simulink model "souk_single_pipeline_4x2"  (R2021a)
settings: Solver=VariableStepAuto  StartTime=0.0  StopTime=10.0  RelTol=1e-3
undefined symbols (not defined in the file): datetime, posixtime
libraries: xbsIndex_r4 x9016, casper_library_misc x75, casper_library_delays x33, casper_library_reorder x22, xps_library x10
(part 35 of 104)

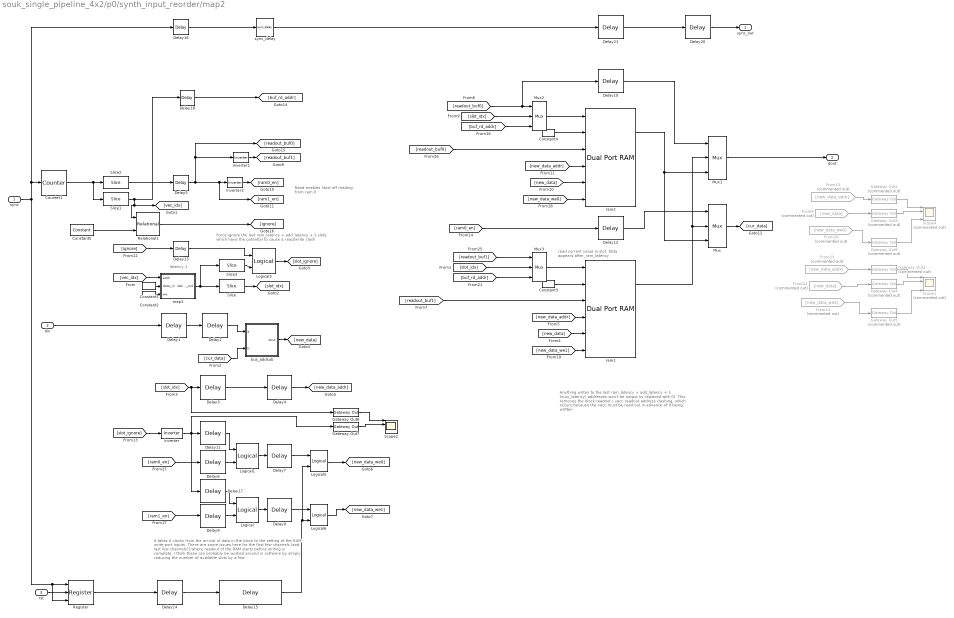
== system souk_single_pipeline_4x2/p0/synth_input_reorder/map2 ==
  note: latency 1
  note: read current value in slot.
      | Data appears after_ram_latency
  note: Read enables
      | Start off reading from ram 0
  note: It takes 6 clocks from the arrival of data in the block
      | to the setting of the RAM write-port inputs. There are some issues
      | here for the first few channels (and last few channels?) where readout
      | of the RAM starts before writing is complete. I think these can probably
      | be worked around in software by simply reducing the number of available
      | slots by a few
  note: Anything writen to the last
      | ram_latency + add_latency + 1 (mux_latency)
      | addresses won't be output (is replaced with 0).
      | This removes the block readout / vacc readout address clashing,
      | which occurs because the vacc must be read out in advance of
      | it being written
  note: Force ignore the last ram_latency + add_latency + 1 slots,
      | which have the potential to cause a read/write clash
  sync : Inport
  din : Inport  Port=2
  rst : Inport  Port=3
  Constant1 : xbsIndex_r4/Constant  const=0  gui_display_data_type=Fixed-point  arith_type=Unsigned  n_bits=32  bin_pt=0  preci_type=Single  exp_width=8  frac_width=24  explicit_period=on  period=1  equ=P=C  opselect=C  inp2=PCIN>>17  opr=+  inp1=P  carry=CIN  dbl_ovrd=off  block_type=constant
  Constant2 : xbsIndex_r4/Constant  const=0  gui_display_data_type=Boolean  arith_type=Boolean  n_bits=32  bin_pt=0  preci_type=Single  exp_width=8  frac_width=24  explicit_period=on  period=1  equ=P=C  opselect=C  inp2=PCIN>>17  opr=+  inp1=P  carry=CIN  dbl_ovrd=off  block_type=constant
  Constant3 : xbsIndex_r4/Constant  const=0  gui_display_data_type=Fixed-point  arith_type=Unsigned  n_bits=2*sample_width * n_samples  bin_pt=0  preci_type=Single  exp_width=8  frac_width=24  explicit_period=on  period=1  equ=P=C  opselect=C  inp2=PCIN>>17  opr=+  inp1=P  carry=CIN  dbl_ovrd=off  block_type=constant
  Constant4 : xbsIndex_r4/Constant  const=0  gui_display_data_type=Fixed-point  arith_type=Unsigned  n_bits=2*sample_width * n_samples  bin_pt=0  preci_type=Single  exp_width=8  frac_width=24  explicit_period=on  period=1  equ=P=C  opselect=C  inp2=PCIN>>17  opr=+  inp1=P  carry=CIN  dbl_ovrd=off  block_type=constant
  Constant5 : xbsIndex_r4/Constant  const="(2^vec_len_bits - 1) - (ram_latency + add_latency +  1 + 1 + 1)"  gui_display_data_type=Fixed-point  arith_type=Unsigned  n_bits=vec_len_bits  bin_pt=0  preci_type=Single  exp_width=8  frac_width=24  explicit_period=on  period=1  equ=P=C  opselect=C  inp2=PCIN>>17  opr=+  inp1=P  carry=CIN  dbl_ovrd=off  block_type=constant
  Counter1 : xbsIndex_r4/Counter  cnt_type=Free Running  cnt_to=Inf  operation=Up  start_count=0  cnt_by_val=1  arith_type=Unsigned  n_bits=vec_len_bits + 1  bin_pt=0  load_pin=off  rst=on  en=off  explicit_period=on  period=1  use_behavioral_HDL=off  implementation=Fabric  dbl_ovrd=off  block_type=counter
  Delay{1,5..6,8,13..14,16,18,20} (9 alike) : xbsIndex_r4/Delay  rst=off  infoeditControl=Selection of Reset will increase slice count due to use of real FFs and instead of SRLs  en=off  latency=1  reg_retiming=on  dbl_ovrd=off  block_type=delay
  Delay10 : xbsIndex_r4/Delay  rst=off  infoeditControl=Selection of Reset will increase slice count due to use of real FFs and instead of SRLs  en=off  latency=ram_latency  reg_retiming=on  dbl_ovrd=off  block_type=delay
  Delay11 : xbsIndex_r4/Delay  rst=off  infoeditControl=Selection of Reset will increase slice count due to use of real FFs and instead of SRLs  en=off  latency=1  reg_retiming=off  dbl_ovrd=off  block_type=delay
  Delay12 : xbsIndex_r4/Delay  rst=off  infoeditControl=Selection of Reset will increase slice count due to use of real FFs and instead of SRLs  en=off  latency=ram_latency  reg_retiming=on  dbl_ovrd=off  block_type=delay
  Delay15 : xbsIndex_r4/Delay  rst=off  infoeditControl=Selection of Reset will increase slice count due to use of real FFs and instead of SRLs  en=off  latency=ram_latency + add_latency +1  reg_retiming=on  dbl_ovrd=off  block_type=delay
  Delay17 : xbsIndex_r4/Delay  rst=off  infoeditControl=Selection of Reset will increase slice count due to use of real FFs and instead of SRLs  en=off  latency=1  reg_retiming=off  dbl_ovrd=off  block_type=delay
  Delay2 : xbsIndex_r4/Delay  rst=off  infoeditControl=Selection of Reset will increase slice count due to use of real FFs and instead of SRLs  en=off  latency=ram_latency+1  reg_retiming=on  dbl_ovrd=off  block_type=delay
  Delay21 : xbsIndex_r4/Delay  rst=off  infoeditControl=Selection of Reset will increase slice count due to use of real FFs and instead of SRLs  en=off  latency=ram_latency  reg_retiming=on  dbl_ovrd=off  block_type=delay
  Delay3 : xbsIndex_r4/Delay  rst=off  infoeditControl=Selection of Reset will increase slice count due to use of real FFs and instead of SRLs  en=off  latency=ram_latency+1  reg_retiming=on  dbl_ovrd=off  block_type=delay
  Delay4 : xbsIndex_r4/Delay  rst=off  infoeditControl=Selection of Reset will increase slice count due to use of real FFs and instead of SRLs  en=off  latency=add_latency  reg_retiming=on  dbl_ovrd=off  block_type=delay
  Delay7 : xbsIndex_r4/Delay  rst=off  infoeditControl=Selection of Reset will increase slice count due to use of real FFs and instead of SRLs  en=off  latency=add_latency  reg_retiming=on  dbl_ovrd=off  block_type=delay
  Delay9 : xbsIndex_r4/Delay  rst=off  infoeditControl=Selection of Reset will increase slice count due to use of real FFs and instead of SRLs  en=off  latency=add_latency  reg_retiming=on  dbl_ovrd=off  block_type=delay
  From15 : From  Commented=on  GotoTag=new_data_addr
  From20 : From  Commented=on  GotoTag=new_data_we0
  From22 : From  Commented=on  GotoTag=new_data
  From23 : From  Commented=on  GotoTag=new_data_addr
  From24 : From  Commented=on  GotoTag=new_data_we1
  From8 : From  Commented=on  GotoTag=new_data
  Gateway Out{1..5,9} (6 alike) : xbsIndex_r4/Gateway Out  Commented=on  inherit_from_input=off  hdl_port=off  rows=1  columns=1  UseAsDAC=off  DACChannel='1'  interface=None  automatic_assignment=on  address_offset=hex2dec('00')  intf_name=''  intf_description=''  timing_constraint=None  locs_specified=off  LOCs={}  io_standard={}  block_type=gatewayout
  Gateway Out6 : xbsIndex_r4/Gateway Out  inherit_from_input=off  hdl_port=off  rows=1  columns=1  UseAsDAC=off  DACChannel='1'  interface=None  automatic_assignment=on  address_offset=hex2dec('00')  intf_name=''  intf_description=''  timing_constraint=None  locs_specified=off  LOCs={}  io_standard={}  block_type=gatewayout
  Gateway Out7 : xbsIndex_r4/Gateway Out  inherit_from_input=off  hdl_port=off  rows=1  columns=1  UseAsDAC=off  DACChannel='1'  interface=None  automatic_assignment=on  address_offset=hex2dec('00')  intf_name=''  intf_description=''  timing_constraint=None  locs_specified=off  LOCs={}  io_standard={}  block_type=gatewayout
  Inverter : xbsIndex_r4/Inverter  en=off  latency=0  dbl_ovrd=off  block_type=inv
  Inverter1 : xbsIndex_r4/Inverter  en=off  latency=0  dbl_ovrd=off  block_type=inv
  Inverter3 : xbsIndex_r4/Inverter  en=off  latency=0  dbl_ovrd=off  block_type=inv
  Logical : xbsIndex_r4/Logical  logical_function=AND  inputs=2  en=off  latency=ram_latency  precision=Full  arith_type=Unsigned  n_bits=16  bin_pt=0  align_bp=on  dbl_ovrd=off  block_type=logical
  Logical1 : xbsIndex_r4/Logical  logical_function=AND  inputs=2  en=off  latency=ram_latency  precision=Full  arith_type=Unsigned  n_bits=16  bin_pt=0  align_bp=on  dbl_ovrd=off  block_type=logical
  Logical3 : xbsIndex_r4/Logical  logical_function=OR  inputs=2  en=off  latency=0  precision=Full  arith_type=Unsigned  n_bits=16  bin_pt=0  align_bp=on  dbl_ovrd=off  block_type=logical
  Logical5 : xbsIndex_r4/Logical  logical_function=AND  inputs=2  en=off  latency=0  precision=Full  arith_type=Unsigned  n_bits=16  bin_pt=0  align_bp=on  dbl_ovrd=off  block_type=logical
  Logical6 : xbsIndex_r4/Logical  logical_function=AND  inputs=2  en=off  latency=0  precision=Full  arith_type=Unsigned  n_bits=16  bin_pt=0  align_bp=on  dbl_ovrd=off  block_type=logical
  Mux : xbsIndex_r4/Mux  inputs=2  en=off  latency=1  precision=Full  arith_type=Unsigned  n_bits=16  bin_pt=14  quantization=Truncate  overflow=Wrap  dbl_ovrd=off  block_type=mux
  Mux1 : xbsIndex_r4/Mux  inputs=2  en=off  latency=1  precision=Full  arith_type=Unsigned  n_bits=16  bin_pt=14  quantization=Truncate  overflow=Wrap  dbl_ovrd=off  block_type=mux
  Mux2 : xbsIndex_r4/Mux  inputs=2  en=off  latency=0  precision=Full  arith_type=Unsigned  n_bits=16  bin_pt=14  quantization=Truncate  overflow=Wrap  dbl_ovrd=off  block_type=mux
  Mux3 : xbsIndex_r4/Mux  inputs=2  en=off  latency=0  precision=Full  arith_type=Unsigned  n_bits=16  bin_pt=14  quantization=Truncate  overflow=Wrap  dbl_ovrd=off  block_type=mux
  Register : xbsIndex_r4/Register  init=0  rst=on  en=on  dbl_ovrd=off  block_type=register
  Relational1 : xbsIndex_r4/Relational  mode=a>b  op_type=Bool  en=off  latency=0  dbl_ovrd=off  block_type=relational
  Scope1 : Scope  Commented=on  NumInputPorts=4
  Scope2 : Scope  NumInputPorts=4
  Scope4 : Scope  Commented=on  NumInputPorts=4
  Slice : xbsIndex_r4/Slice  nbits=vec_len_bits  boolean_output=off  mode=Lower Bit Location + Width  bit1=0  base1=MSB of Input  bit0=0  base0=LSB of Input  dbl_ovrd=off  block_type=slice
  Slice1 : xbsIndex_r4/Slice  nbits=vec_len_bits  boolean_output=off  mode=Lower Bit Location + Width  bit1=0  base1=MSB of Input  bit0=0  base0=LSB of Input  dbl_ovrd=off  block_type=slice
  Slice2 : xbsIndex_r4/Slice  nbits=1  boolean_output=on  mode=Lower Bit Location + Width  bit1=0  base1=MSB of Input  bit0=vec_len_bits  base0=LSB of Input  dbl_ovrd=off  block_type=slice
  Slice3 : xbsIndex_r4/Slice  nbits=1  boolean_output=on  mode=Upper Bit Location + Width  bit1=0  base1=MSB of Input  bit0=0  base0=LSB of Input  dbl_ovrd=off  block_type=slice
  bus_addsub : Subsystem  AncestorBlock=casper_library_bus/bus_addsub  mask(bus_addsub){opmode=0, n_bits_a=sample_width*ones(n_samples,1), bin_pt_a=zeros(n_samples,1), type_a=1, n_bits_b=sample_width*ones(n_samples,1), bin_pt_b=zeros(n_samples,1), type_b=1, cmplx=on, misc=off, async=off, floating_point=off, float_type=single, exp_width=6, frac_width=19, n_bits_out=sample_width*ones(n_samples,1), bin_pt_out=zeros(n_samples,1), type_out=1, quantization=0, overflow=1, add_implementation=behavioral HDL, csp_latency=add_latency, pipeline_en=off, pipeline_latency=0}
      mask prompts: opmode "mode (Addition=0, Subtraction=1)"; n_bits_a "a input bit widths"; bin_pt_a "a input binary points"; type_a "a input type (Unsigned=0, Signed=1)"; n_bits_b "b input bit widths"; bin_pt_b "b input binary points"; type_b "b input type (Unsigned=0, Signed=1)"; cmplx "complex"; misc "misc support"; async "asynchronous operation"; floating_point "floating point"; exp_width "exponent width"; frac_width "fraction width"; n_bits_out "output bit widths"; bin_pt_out "output binary points"; type_out "output type (Unsigned=0, Signed=1)"; quantization "quantization strategy (Truncate=0, Round  (unbiased: +/- Inf)=1)"; overflow "overflow strategy (Wrap=0, Saturate=1, Flag as error=2)"; add_implementation "adder implementation"; csp_latency "latency"; pipeline_en "pipeline enable"; pipeline_latency "pipeline latency"
      mask help: Add/subtract components of two busses
      mask init: same as souk_single_pipeline_4x2/p0/bus_addsub
      mask Callback floating_point:
      | onoff = get_param(gcb, 'floating_point');
      | if strcmp(onoff,'on')
      |     enable_fixpt = 'off';
      |     set_param_state(gcb, 'float_type', 'on')
      | 
      |     f_type = get_param(gcb, 'float_type');
      |     if strcmp(f_type,'custom')
      |         set_param_state(gcb, 'exp_width', 'on')
      |         set_param_state(gcb, 'frac_width', 'on')
      |     else
      |         set_param_state(gcb, 'exp_width', 'off')
      |         set_param_state(gcb, 'frac_width', 'off')
      |     end
      | 
      | 
      | else
      |     enable_fixpt = 'on';
      |     set_param_state(gcb, 'float_type', 'off')
      |     set_param_state(gcb, 'exp_width', 'off')
      |     set_param_state(gcb, 'frac_width', 'off')
      | end
      | 
      | set_param_state(gcb, 'n_bits_a', enable_fixpt)
      | set_param_state(gcb, 'bin_pt_a', enable_fixpt)
      | set_param_state(gcb, 'type_a', enable_fixpt)
      | set_param_state(gcb, 'n_bits_b', enable_fixpt)
      | set_param_state(gcb, 'bin_pt_b', enable_fixpt)
      | set_param_state(gcb, 'type_b', enable_fixpt)
      | 
      | set_param_state(gcb, 'n_bits_out', enable_fixpt)
      | set_param_state(gcb, 'bin_pt_out', enable_fixpt)
      | set_param_state(gcb, 'type_out', enable_fixpt)
      | set_param_state(gcb, 'quantization', enable_fixpt)
      | set_param_state(gcb, 'overflow', enable_fixpt)
      mask TypeOptions float_type: single | custom
      mask Callback float_type:
      | f_type = get_param(gcb, 'float_type');
      | if strcmp(f_type,'custom')
      |     set_param_state(gcb, 'exp_width', 'on')
      |     set_param_state(gcb, 'frac_width', 'on')
      | else
      |     set_param_state(gcb, 'exp_width', 'off')
      |     set_param_state(gcb, 'frac_width', 'off')
      | end
      mask TypeOptions add_implementation: behavioral HDL | fabric core | DSP48 core
  map1 : Subsystem  Tag=xps:bram  AncestorBlock=xps_library/Memory/shared_bram  mask{arith_type=Unsigned, addr_width=vec_len_bits, data_width=16, reg_prim_output=off, reg_core_output=off, optimization=Minimum_Area, data_bin_pt=0, init_vals=[2^vec_len_bits-1:-1:0], sample_rate=1, desc_str="", type_desc='uint32'}
      mask prompts: arith_type "Output Data Type"; addr_width "Address width"; data_width "Data Width"; reg_prim_output "Register Primitive Output"; reg_core_output "Register Core Output"; data_bin_pt "Data Binary Point"; init_vals "Initial values (simulation only)"; sample_rate "Sample rate"; desc_str "Description"; type_desc "Data Type Description"
      mask init:
      | shared_bram_mask;
      mask TypeOptions arith_type: Unsigned | Signed  (2's comp)
      mask TypeOptions data_width: 8 | 16 | 32 | 64 | 128 | 256 | 512 | 1024
      mask TypeOptions optimization: Minimum_Area | Low_Power
  ram1 : xbsIndex_r4/Dual Port RAM  depth=2^vec_len_bits  initVector=zeros(1,2^vec_len_bits)  distributed_mem=Block RAM  init_a=0  init_b=0  rst_a=off  rst_b=off  en_a=off  en_b=off  latency=ram_latency  write_mode_A=Read Before Write  write_mode_B=Read Before Write  optimize=Area  dbl_ovrd=off  simulation_type=fast_sim  block_type=dpram
  ram2 : xbsIndex_r4/Dual Port RAM  depth=2^vec_len_bits  initVector=zeros(1,2^vec_len_bits)  distributed_mem=Block RAM  init_a=0  init_b=0  rst_a=off  rst_b=off  en_a=off  en_b=off  latency=ram_latency  write_mode_A=Read Before Write  write_mode_B=Read Before Write  optimize=Area  dbl_ovrd=off  simulation_type=fast_sim  block_type=dpram
  sync_delay : casper_library_delays/sync_delay  DelayLen=2^vec_len_bits
      settings: SourceProductName=CASPER DSP Blockset
  sync_out : Outport
  dout : Outport  Port=2
  wires:
  [readout_buf1] -> Mux3/1
  Delay10/1 -> Mux1/1
  [readout_buf0] -> Mux2/1, Delay10/1
  Delay5/1 -> Inverter1/1, [readout_buf0], [ram1_en], Inverter3/1
  Delay15/1 -> Logical6/2, Logical5/2
  Logical6/1 -> [new_data_we1]
  Delay9/1 -> Logical6/1
  Logical5/1 -> [new_data_we0]
  Delay7/1 -> Logical5/1
  Delay14/1 -> Delay15/1
  Register/1 -> Delay14/1
  rst/1 -> Register/2
  Gateway Out6/1 -> Scope2/1
  Gateway Out7/1 -> Scope2/2
  [slot_idx] -> Delay3/1, Gateway Out6/1
  Delay13/1 -> Logical3/1
  From24/1 -> Gateway Out5/1
  From22/1 -> Gateway Out4/1
  From23/1 -> Gateway Out2/1
  Gateway Out5/1 -> Scope1/4
  Gateway Out4/1 -> Scope1/2
  ? -> Scope1/3
  Gateway Out2/1 -> Scope1/1
  Slice3/1 -> Logical3/2
  [ignore] -> Delay13/1
  Logical3/1 -> [slot_ignore]
  Logical1/1 -> Delay7/1
  Delay11/1 -> Logical1/1
  Delay6/1 -> Logical1/2
  Delay17/1 -> Logical/1
  Logical/1 -> Delay9/1
  Delay8/1 -> Logical/2
  Inverter/1 -> Delay11/1, Delay17/1, Gateway Out7/1
  [slot_ignore] -> Inverter/1
  [new_data] -> ram2/5
  [new_data_we0] -> ram2/6
  [new_data_addr] -> ram2/4
  sync/1 -> Delay16/1, Counter1/1, Register/1, Register/3
  sync_delay/1 -> Delay21/1
  Delay21/1 -> Delay20/1
  Delay20/1 -> sync_out/1
  Mux1/1 -> dout/1
  [readout_buf1] -> ram1/3
  Delay12/1 -> Mux/1
  [ram0_en] -> Delay12/1
  [new_data_we1] -> ram1/6
  [new_data_addr] -> ram1/4
  [new_data] -> ram1/5
  [ram1_en] -> Delay8/1
  [ram0_en] -> Delay6/1
  ram1/1 -> Mux/2, Mux1/2
  Constant4/1 -> ram2/2
  Constant3/1 -> ram1/2
  Mux3/1 -> ram1/1
  [buf_rd_addr] -> Mux3/3
  [slot_idx] -> Mux3/2
  [slot_idx] -> Mux2/2
  [buf_rd_addr] -> Mux2/3
  Mux2/1 -> ram2/1
  Mux/1 -> [cur_data]
  [readout_buf0] -> ram2/3
  ram2/1 -> Mux1/3, Mux/3
  Slice2/1 -> Delay5/1
  Delay4/1 -> [new_data_addr]
  bus_addsub/1(dout) -> [new_data]
  Delay3/1 -> Delay4/1
  Delay2/1 -> bus_addsub/1(a)
  [cur_data] -> bus_addsub/2(b)
  Delay1/1 -> Delay2/1
  Slice/1 -> [slot_idx]
  din/1 -> Delay1/1
  Constant2/1 -> map1/3(we)
  Constant1/1 -> map1/2(data_in)
  [vec_idx] -> map1/1(addr)
  Slice1/1 -> Delay18/1, Relational1/1, [vec_idx]
  Counter1/1 -> Slice1/1, Slice2/1
  map1/1(data_out) -> Slice/1, Slice3/1
  Inverter3/1 -> [ram0_en]
  Constant5/1 -> Relational1/2
  Relational1/1 -> [ignore]
  Inverter1/1 -> [readout_buf1]
  Delay16/1 -> sync_delay/1
  Gateway Out1/1 -> Scope4/1
  ? -> Scope4/3
  Gateway Out3/1 -> Scope4/2
  Gateway Out9/1 -> Scope4/4
  From15/1 -> Gateway Out1/1
  From8/1 -> Gateway Out3/1
  From20/1 -> Gateway Out9/1
  Delay18/1 -> [buf_rd_addr]

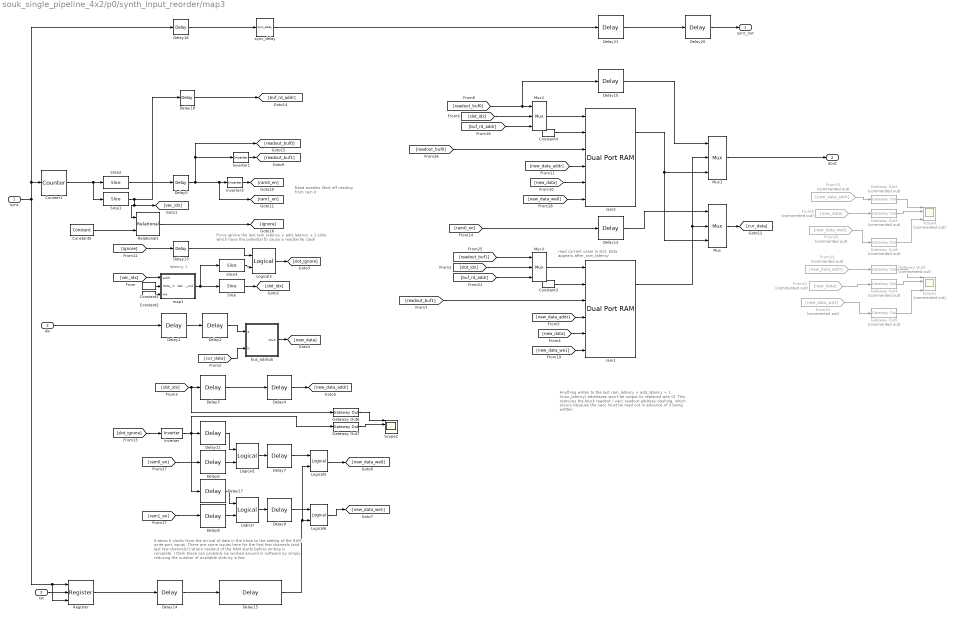
== system souk_single_pipeline_4x2/p0/synth_input_reorder/map3 ==
  note: Force ignore the last ram_latency + add_latency + 1 slots,
      | which have the potential to cause a read/write clash
  note: Anything writen to the last
      | ram_latency + add_latency + 1 (mux_latency)
      | addresses won't be output (is replaced with 0).
      | This removes the block readout / vacc readout address clashing,
      | which occurs because the vacc must be read out in advance of
      | it being written
  note: It takes 6 clocks from the arrival of data in the block
      | to the setting of the RAM write-port inputs. There are some issues
      | here for the first few channels (and last few channels?) where readout
      | of the RAM starts before writing is complete. I think these can probably
      | be worked around in software by simply reducing the number of available
      | slots by a few
  note: Read enables
      | Start off reading from ram 0
  note: read current value in slot.
      | Data appears after_ram_latency
  note: latency 1
  sync : Inport
  din : Inport  Port=2
  rst : Inport  Port=3
  Constant1 : xbsIndex_r4/Constant  const=0  gui_display_data_type=Fixed-point  arith_type=Unsigned  n_bits=32  bin_pt=0  preci_type=Single  exp_width=8  frac_width=24  explicit_period=on  period=1  equ=P=C  opselect=C  inp2=PCIN>>17  opr=+  inp1=P  carry=CIN  dbl_ovrd=off  block_type=constant
  Constant2 : xbsIndex_r4/Constant  const=0  gui_display_data_type=Boolean  arith_type=Boolean  n_bits=32  bin_pt=0  preci_type=Single  exp_width=8  frac_width=24  explicit_period=on  period=1  equ=P=C  opselect=C  inp2=PCIN>>17  opr=+  inp1=P  carry=CIN  dbl_ovrd=off  block_type=constant
  Constant3 : xbsIndex_r4/Constant  const=0  gui_display_data_type=Fixed-point  arith_type=Unsigned  n_bits=2*sample_width * n_samples  bin_pt=0  preci_type=Single  exp_width=8  frac_width=24  explicit_period=on  period=1  equ=P=C  opselect=C  inp2=PCIN>>17  opr=+  inp1=P  carry=CIN  dbl_ovrd=off  block_type=constant
  Constant4 : xbsIndex_r4/Constant  const=0  gui_display_data_type=Fixed-point  arith_type=Unsigned  n_bits=2*sample_width * n_samples  bin_pt=0  preci_type=Single  exp_width=8  frac_width=24  explicit_period=on  period=1  equ=P=C  opselect=C  inp2=PCIN>>17  opr=+  inp1=P  carry=CIN  dbl_ovrd=off  block_type=constant
  Constant5 : xbsIndex_r4/Constant  const="(2^vec_len_bits - 1) - (ram_latency + add_latency +  1 + 1 + 1)"  gui_display_data_type=Fixed-point  arith_type=Unsigned  n_bits=vec_len_bits  bin_pt=0  preci_type=Single  exp_width=8  frac_width=24  explicit_period=on  period=1  equ=P=C  opselect=C  inp2=PCIN>>17  opr=+  inp1=P  carry=CIN  dbl_ovrd=off  block_type=constant
  Counter1 : xbsIndex_r4/Counter  cnt_type=Free Running  cnt_to=Inf  operation=Up  start_count=0  cnt_by_val=1  arith_type=Unsigned  n_bits=vec_len_bits + 1  bin_pt=0  load_pin=off  rst=on  en=off  explicit_period=on  period=1  use_behavioral_HDL=off  implementation=Fabric  dbl_ovrd=off  block_type=counter
  Delay{1,5..6,8,13..14,16,18,20} (9 alike) : xbsIndex_r4/Delay  rst=off  infoeditControl=Selection of Reset will increase slice count due to use of real FFs and instead of SRLs  en=off  latency=1  reg_retiming=on  dbl_ovrd=off  block_type=delay
  Delay10 : xbsIndex_r4/Delay  rst=off  infoeditControl=Selection of Reset will increase slice count due to use of real FFs and instead of SRLs  en=off  latency=ram_latency  reg_retiming=on  dbl_ovrd=off  block_type=delay
  Delay11 : xbsIndex_r4/Delay  rst=off  infoeditControl=Selection of Reset will increase slice count due to use of real FFs and instead of SRLs  en=off  latency=1  reg_retiming=off  dbl_ovrd=off  block_type=delay
  Delay12 : xbsIndex_r4/Delay  rst=off  infoeditControl=Selection of Reset will increase slice count due to use of real FFs and instead of SRLs  en=off  latency=ram_latency  reg_retiming=on  dbl_ovrd=off  block_type=delay
  Delay15 : xbsIndex_r4/Delay  rst=off  infoeditControl=Selection of Reset will increase slice count due to use of real FFs and instead of SRLs  en=off  latency=ram_latency + add_latency +1  reg_retiming=on  dbl_ovrd=off  block_type=delay
  Delay17 : xbsIndex_r4/Delay  rst=off  infoeditControl=Selection of Reset will increase slice count due to use of real FFs and instead of SRLs  en=off  latency=1  reg_retiming=off  dbl_ovrd=off  block_type=delay
  Delay2 : xbsIndex_r4/Delay  rst=off  infoeditControl=Selection of Reset will increase slice count due to use of real FFs and instead of SRLs  en=off  latency=ram_latency+1  reg_retiming=on  dbl_ovrd=off  block_type=delay
  Delay21 : xbsIndex_r4/Delay  rst=off  infoeditControl=Selection of Reset will increase slice count due to use of real FFs and instead of SRLs  en=off  latency=ram_latency  reg_retiming=on  dbl_ovrd=off  block_type=delay
  Delay3 : xbsIndex_r4/Delay  rst=off  infoeditControl=Selection of Reset will increase slice count due to use of real FFs and instead of SRLs  en=off  latency=ram_latency+1  reg_retiming=on  dbl_ovrd=off  block_type=delay
  Delay4 : xbsIndex_r4/Delay  rst=off  infoeditControl=Selection of Reset will increase slice count due to use of real FFs and instead of SRLs  en=off  latency=add_latency  reg_retiming=on  dbl_ovrd=off  block_type=delay
  Delay7 : xbsIndex_r4/Delay  rst=off  infoeditControl=Selection of Reset will increase slice count due to use of real FFs and instead of SRLs  en=off  latency=add_latency  reg_retiming=on  dbl_ovrd=off  block_type=delay
  Delay9 : xbsIndex_r4/Delay  rst=off  infoeditControl=Selection of Reset will increase slice count due to use of real FFs and instead of SRLs  en=off  latency=add_latency  reg_retiming=on  dbl_ovrd=off  block_type=delay
  From15 : From  Commented=on  GotoTag=new_data_addr
  From20 : From  Commented=on  GotoTag=new_data_we0
  From22 : From  Commented=on  GotoTag=new_data
  From23 : From  Commented=on  GotoTag=new_data_addr
  From24 : From  Commented=on  GotoTag=new_data_we1
  From8 : From  Commented=on  GotoTag=new_data
  Gateway Out{1..5,9} (6 alike) : xbsIndex_r4/Gateway Out  Commented=on  inherit_from_input=off  hdl_port=off  rows=1  columns=1  UseAsDAC=off  DACChannel='1'  interface=None  automatic_assignment=on  address_offset=hex2dec('00')  intf_name=''  intf_description=''  timing_constraint=None  locs_specified=off  LOCs={}  io_standard={}  block_type=gatewayout
  Gateway Out6 : xbsIndex_r4/Gateway Out  inherit_from_input=off  hdl_port=off  rows=1  columns=1  UseAsDAC=off  DACChannel='1'  interface=None  automatic_assignment=on  address_offset=hex2dec('00')  intf_name=''  intf_description=''  timing_constraint=None  locs_specified=off  LOCs={}  io_standard={}  block_type=gatewayout
  Gateway Out7 : xbsIndex_r4/Gateway Out  inherit_from_input=off  hdl_port=off  rows=1  columns=1  UseAsDAC=off  DACChannel='1'  interface=None  automatic_assignment=on  address_offset=hex2dec('00')  intf_name=''  intf_description=''  timing_constraint=None  locs_specified=off  LOCs={}  io_standard={}  block_type=gatewayout
  Inverter : xbsIndex_r4/Inverter  en=off  latency=0  dbl_ovrd=off  block_type=inv
  Inverter1 : xbsIndex_r4/Inverter  en=off  latency=0  dbl_ovrd=off  block_type=inv
  Inverter3 : xbsIndex_r4/Inverter  en=off  latency=0  dbl_ovrd=off  block_type=inv
  Logical : xbsIndex_r4/Logical  logical_function=AND  inputs=2  en=off  latency=ram_latency  precision=Full  arith_type=Unsigned  n_bits=16  bin_pt=0  align_bp=on  dbl_ovrd=off  block_type=logical
  Logical1 : xbsIndex_r4/Logical  logical_function=AND  inputs=2  en=off  latency=ram_latency  precision=Full  arith_type=Unsigned  n_bits=16  bin_pt=0  align_bp=on  dbl_ovrd=off  block_type=logical
  Logical3 : xbsIndex_r4/Logical  logical_function=OR  inputs=2  en=off  latency=0  precision=Full  arith_type=Unsigned  n_bits=16  bin_pt=0  align_bp=on  dbl_ovrd=off  block_type=logical
  Logical5 : xbsIndex_r4/Logical  logical_function=AND  inputs=2  en=off  latency=0  precision=Full  arith_type=Unsigned  n_bits=16  bin_pt=0  align_bp=on  dbl_ovrd=off  block_type=logical
  Logical6 : xbsIndex_r4/Logical  logical_function=AND  inputs=2  en=off  latency=0  precision=Full  arith_type=Unsigned  n_bits=16  bin_pt=0  align_bp=on  dbl_ovrd=off  block_type=logical
  Mux : xbsIndex_r4/Mux  inputs=2  en=off  latency=1  precision=Full  arith_type=Unsigned  n_bits=16  bin_pt=14  quantization=Truncate  overflow=Wrap  dbl_ovrd=off  block_type=mux
  Mux1 : xbsIndex_r4/Mux  inputs=2  en=off  latency=1  precision=Full  arith_type=Unsigned  n_bits=16  bin_pt=14  quantization=Truncate  overflow=Wrap  dbl_ovrd=off  block_type=mux
  Mux2 : xbsIndex_r4/Mux  inputs=2  en=off  latency=0  precision=Full  arith_type=Unsigned  n_bits=16  bin_pt=14  quantization=Truncate  overflow=Wrap  dbl_ovrd=off  block_type=mux
  Mux3 : xbsIndex_r4/Mux  inputs=2  en=off  latency=0  precision=Full  arith_type=Unsigned  n_bits=16  bin_pt=14  quantization=Truncate  overflow=Wrap  dbl_ovrd=off  block_type=mux
  Register : xbsIndex_r4/Register  init=0  rst=on  en=on  dbl_ovrd=off  block_type=register
  Relational1 : xbsIndex_r4/Relational  mode=a>b  op_type=Bool  en=off  latency=0  dbl_ovrd=off  block_type=relational
  Scope1 : Scope  Commented=on  NumInputPorts=4
  Scope2 : Scope  NumInputPorts=4
  Scope4 : Scope  Commented=on  NumInputPorts=4
  Slice : xbsIndex_r4/Slice  nbits=vec_len_bits  boolean_output=off  mode=Lower Bit Location + Width  bit1=0  base1=MSB of Input  bit0=0  base0=LSB of Input  dbl_ovrd=off  block_type=slice
  Slice1 : xbsIndex_r4/Slice  nbits=vec_len_bits  boolean_output=off  mode=Lower Bit Location + Width  bit1=0  base1=MSB of Input  bit0=0  base0=LSB of Input  dbl_ovrd=off  block_type=slice
  Slice2 : xbsIndex_r4/Slice  nbits=1  boolean_output=on  mode=Lower Bit Location + Width  bit1=0  base1=MSB of Input  bit0=vec_len_bits  base0=LSB of Input  dbl_ovrd=off  block_type=slice
  Slice3 : xbsIndex_r4/Slice  nbits=1  boolean_output=on  mode=Upper Bit Location + Width  bit1=0  base1=MSB of Input  bit0=0  base0=LSB of Input  dbl_ovrd=off  block_type=slice
  bus_addsub : Subsystem  AncestorBlock=casper_library_bus/bus_addsub  mask(bus_addsub){opmode=0, n_bits_a=sample_width*ones(n_samples,1), bin_pt_a=zeros(n_samples,1), type_a=1, n_bits_b=sample_width*ones(n_samples,1), bin_pt_b=zeros(n_samples,1), type_b=1, cmplx=on, misc=off, async=off, floating_point=off, float_type=single, exp_width=6, frac_width=19, n_bits_out=sample_width*ones(n_samples,1), bin_pt_out=zeros(n_samples,1), type_out=1, quantization=0, overflow=1, add_implementation=behavioral HDL, csp_latency=add_latency, pipeline_en=off, pipeline_latency=0}
      mask prompts: opmode "mode (Addition=0, Subtraction=1)"; n_bits_a "a input bit widths"; bin_pt_a "a input binary points"; type_a "a input type (Unsigned=0, Signed=1)"; n_bits_b "b input bit widths"; bin_pt_b "b input binary points"; type_b "b input type (Unsigned=0, Signed=1)"; cmplx "complex"; misc "misc support"; async "asynchronous operation"; floating_point "floating point"; exp_width "exponent width"; frac_width "fraction width"; n_bits_out "output bit widths"; bin_pt_out "output binary points"; type_out "output type (Unsigned=0, Signed=1)"; quantization "quantization strategy (Truncate=0, Round  (unbiased: +/- Inf)=1)"; overflow "overflow strategy (Wrap=0, Saturate=1, Flag as error=2)"; add_implementation "adder implementation"; csp_latency "latency"; pipeline_en "pipeline enable"; pipeline_latency "pipeline latency"
      mask help: Add/subtract components of two busses
      mask init: same as souk_single_pipeline_4x2/p0/bus_addsub
      mask Callback floating_point:
      | onoff = get_param(gcb, 'floating_point');
      | if strcmp(onoff,'on')
      |     enable_fixpt = 'off';
      |     set_param_state(gcb, 'float_type', 'on')
      | 
      |     f_type = get_param(gcb, 'float_type');
      |     if strcmp(f_type,'custom')
      |         set_param_state(gcb, 'exp_width', 'on')
      |         set_param_state(gcb, 'frac_width', 'on')
      |     else
      |         set_param_state(gcb, 'exp_width', 'off')
      |         set_param_state(gcb, 'frac_width', 'off')
      |     end
      | 
      | 
      | else
      |     enable_fixpt = 'on';
      |     set_param_state(gcb, 'float_type', 'off')
      |     set_param_state(gcb, 'exp_width', 'off')
      |     set_param_state(gcb, 'frac_width', 'off')
      | end
      | 
      | set_param_state(gcb, 'n_bits_a', enable_fixpt)
      | set_param_state(gcb, 'bin_pt_a', enable_fixpt)
      | set_param_state(gcb, 'type_a', enable_fixpt)
      | set_param_state(gcb, 'n_bits_b', enable_fixpt)
      | set_param_state(gcb, 'bin_pt_b', enable_fixpt)
      | set_param_state(gcb, 'type_b', enable_fixpt)
      | 
      | set_param_state(gcb, 'n_bits_out', enable_fixpt)
      | set_param_state(gcb, 'bin_pt_out', enable_fixpt)
      | set_param_state(gcb, 'type_out', enable_fixpt)
      | set_param_state(gcb, 'quantization', enable_fixpt)
      | set_param_state(gcb, 'overflow', enable_fixpt)
      mask TypeOptions float_type: single | custom
      mask Callback float_type:
      | f_type = get_param(gcb, 'float_type');
      | if strcmp(f_type,'custom')
      |     set_param_state(gcb, 'exp_width', 'on')
      |     set_param_state(gcb, 'frac_width', 'on')
      | else
      |     set_param_state(gcb, 'exp_width', 'off')
      |     set_param_state(gcb, 'frac_width', 'off')
      | end
      mask TypeOptions add_implementation: behavioral HDL | fabric core | DSP48 core
  map1 : Subsystem  Tag=xps:bram  AncestorBlock=xps_library/Memory/shared_bram  mask{arith_type=Unsigned, addr_width=vec_len_bits, data_width=16, reg_prim_output=off, reg_core_output=off, optimization=Minimum_Area, data_bin_pt=0, init_vals=[2^vec_len_bits-1:-1:0], sample_rate=1, desc_str="", type_desc='uint32'}
      mask prompts: arith_type "Output Data Type"; addr_width "Address width"; data_width "Data Width"; reg_prim_output "Register Primitive Output"; reg_core_output "Register Core Output"; data_bin_pt "Data Binary Point"; init_vals "Initial values (simulation only)"; sample_rate "Sample rate"; desc_str "Description"; type_desc "Data Type Description"
      mask init:
      | shared_bram_mask;
      mask TypeOptions arith_type: Unsigned | Signed  (2's comp)
      mask TypeOptions data_width: 8 | 16 | 32 | 64 | 128 | 256 | 512 | 1024
      mask TypeOptions optimization: Minimum_Area | Low_Power
  ram1 : xbsIndex_r4/Dual Port RAM  depth=2^vec_len_bits  initVector=zeros(1,2^vec_len_bits)  distributed_mem=Block RAM  init_a=0  init_b=0  rst_a=off  rst_b=off  en_a=off  en_b=off  latency=ram_latency  write_mode_A=Read Before Write  write_mode_B=Read Before Write  optimize=Area  dbl_ovrd=off  simulation_type=fast_sim  block_type=dpram
  ram2 : xbsIndex_r4/Dual Port RAM  depth=2^vec_len_bits  initVector=zeros(1,2^vec_len_bits)  distributed_mem=Block RAM  init_a=0  init_b=0  rst_a=off  rst_b=off  en_a=off  en_b=off  latency=ram_latency  write_mode_A=Read Before Write  write_mode_B=Read Before Write  optimize=Area  dbl_ovrd=off  simulation_type=fast_sim  block_type=dpram
  sync_delay : casper_library_delays/sync_delay  DelayLen=2^vec_len_bits
      settings: SourceProductName=CASPER DSP Blockset
  sync_out : Outport
  dout : Outport  Port=2
  wires:
  Delay18/1 -> [buf_rd_addr]
  From20/1 -> Gateway Out9/1
  From8/1 -> Gateway Out3/1
  From15/1 -> Gateway Out1/1
  Gateway Out9/1 -> Scope4/4
  Gateway Out3/1 -> Scope4/2
  ? -> Scope4/3
  Gateway Out1/1 -> Scope4/1
  Delay16/1 -> sync_delay/1
  Inverter1/1 -> [readout_buf1]
  Relational1/1 -> [ignore]
  Constant5/1 -> Relational1/2
  Inverter3/1 -> [ram0_en]
  map1/1(data_out) -> Slice3/1, Slice/1
  Counter1/1 -> Slice2/1, Slice1/1
  Slice1/1 -> [vec_idx], Relational1/1, Delay18/1
  [vec_idx] -> map1/1(addr)
  Constant1/1 -> map1/2(data_in)
  Constant2/1 -> map1/3(we)
  din/1 -> Delay1/1
  Slice/1 -> [slot_idx]
  Delay1/1 -> Delay2/1
  [cur_data] -> bus_addsub/2(b)
  Delay2/1 -> bus_addsub/1(a)
  Delay3/1 -> Delay4/1
  bus_addsub/1(dout) -> [new_data]
  Delay4/1 -> [new_data_addr]
  Slice2/1 -> Delay5/1
  ram2/1 -> Mux/3, Mux1/3
  [readout_buf0] -> ram2/3
  Mux/1 -> [cur_data]
  Mux2/1 -> ram2/1
  [buf_rd_addr] -> Mux2/3
  [slot_idx] -> Mux2/2
  [slot_idx] -> Mux3/2
  [buf_rd_addr] -> Mux3/3
  Mux3/1 -> ram1/1
  Constant3/1 -> ram1/2
  Constant4/1 -> ram2/2
  ram1/1 -> Mux1/2, Mux/2
  [ram0_en] -> Delay6/1
  [ram1_en] -> Delay8/1
  [new_data] -> ram1/5
  [new_data_addr] -> ram1/4
  [new_data_we1] -> ram1/6
  [ram0_en] -> Delay12/1
  Delay12/1 -> Mux/1
  [readout_buf1] -> ram1/3
  Mux1/1 -> dout/1
  Delay20/1 -> sync_out/1
  Delay21/1 -> Delay20/1
  sync_delay/1 -> Delay21/1
  sync/1 -> Register/3, Register/1, Counter1/1, Delay16/1
  [new_data_addr] -> ram2/4
  [new_data_we0] -> ram2/6
  [new_data] -> ram2/5
  [slot_ignore] -> Inverter/1
  Inverter/1 -> Gateway Out7/1, Delay17/1, Delay11/1
  Delay8/1 -> Logical/2
  Logical/1 -> Delay9/1
  Delay17/1 -> Logical/1
  Delay6/1 -> Logical1/2
  Delay11/1 -> Logical1/1
  Logical1/1 -> Delay7/1
  Logical3/1 -> [slot_ignore]
  [ignore] -> Delay13/1
  Slice3/1 -> Logical3/2
  Gateway Out2/1 -> Scope1/1
  ? -> Scope1/3
  Gateway Out4/1 -> Scope1/2
  Gateway Out5/1 -> Scope1/4
  From23/1 -> Gateway Out2/1
  From22/1 -> Gateway Out4/1
  From24/1 -> Gateway Out5/1
  Delay13/1 -> Logical3/1
  [slot_idx] -> Gateway Out6/1, Delay3/1
  Gateway Out7/1 -> Scope2/2
  Gateway Out6/1 -> Scope2/1
  rst/1 -> Register/2
  Register/1 -> Delay14/1
  Delay14/1 -> Delay15/1
  Delay7/1 -> Logical5/1
  Logical5/1 -> [new_data_we0]
  Delay9/1 -> Logical6/1
  Logical6/1 -> [new_data_we1]
  Delay15/1 -> Logical5/2, Logical6/2
  Delay5/1 -> Inverter3/1, [ram1_en], [readout_buf0], Inverter1/1
  [readout_buf0] -> Delay10/1, Mux2/1
  Delay10/1 -> Mux1/1
  [readout_buf1] -> Mux3/1

== system souk_single_pipeline_4x2/p0/synth_input_reorder/munge1 ==
  din : Inport
  join : Subsystem  AncestorBlock=casper_library_flow_control/bus_create  mask(bus_create){inputNum=16}
      mask prompts: inputNum "Number of inputs:"
      mask init:
      | bus_create_init(gcb,...
      |     'inputNum', inputNum);
  reinterpret : xbsIndex_r4/Reinterpret  force_arith_type=on  arith_type=Unsigned  force_bin_pt=on  bin_pt=0  block_type=reinterpret
  reinterpret_out : xbsIndex_r4/Reinterpret  force_arith_type=on  arith_type=Unsigned  force_bin_pt=on  bin_pt=0  block_type=reinterpret
  split : Subsystem  AncestorBlock=casper_library_flow_control/bus_expand  mask(bus_expand){mode=divisions of arbitrary size, outputNum=16, outputWidth=[36;36;36;36;36;36;36;36;36;36;36;36;36;36;36;36], outputBinaryPt=[0 0 0 0 0 0 0 0 0 0 0 0 0 0 0 0], outputArithmeticType=[0 0 0 0 0 0 0 0 0 0 0 0 0 0 0 0], show_format=off, outputToWorkspace=off, variablePrefix=out, outputToModelAsWell=on}
      mask prompts: outputNum "Number of outputs:"; outputWidth "Output width:"; outputBinaryPt "Output binary point position:"; outputArithmeticType "Output arithmetic type (ufix=0, fix=1, bool=2):"; show_format "Print format string?"; outputToWorkspace "Output to workspace?"; variablePrefix "Variable name prefix:"; outputToModelAsWell "Output to model as well?"
      mask help:
      | Expands a 'bus' made using a bus_create or Xilinx
      | concat block.
      | The input will be divided into the specified number
      | of outputs with the specified arithmetic types.
      | Divisions are made from most significant bit.
      mask init: same as souk_single_pipeline_4x2/bus_expand
      settings: AttributesFormatString=16 outputs
      mask TypeOptions mode: divisions of equal size | divisions of arbitrary size
      mask Callback mode: %bus_expand_callback();
      mask Callback outputWidth: %bus_expand_callback();
      mask Callback outputToWorkspace: %bus_expand_callback();
  dout : Outport
  wires:
  split/16(lsb_out1) -> join/16(in16)
  split/14(out3) -> join/15(in15)
  split/12(out5) -> join/14(in14)
  split/10(out7) -> join/13(in13)
  split/8(out9) -> join/12(in12)
  split/6(out11) -> join/11(in11)
  split/4(out13) -> join/10(in10)
  split/2(out15) -> join/9(in9)
  split/15(out2) -> join/8(in8)
  split/13(out4) -> join/7(in7)
  split/11(out6) -> join/6(in6)
  split/9(out8) -> join/5(in5)
  split/7(out10) -> join/4(in4)
  split/5(out12) -> join/3(in3)
  split/3(out14) -> join/2(in2)
  split/1(msb_out16) -> join/1(in1)
  join/1(bus_out) -> reinterpret_out/1
  reinterpret/1 -> split/1(bus_in)
  din/1 -> reinterpret/1
  reinterpret_out/1 -> dout/1
